simulink library "ece3413"  (R2018b)
settings: Solver=VariableStepAuto  StartTime=0.0  StopTime=10.0  RelTol=1e-3
settings Model: Creator=lbai  LastModifiedBy=bai

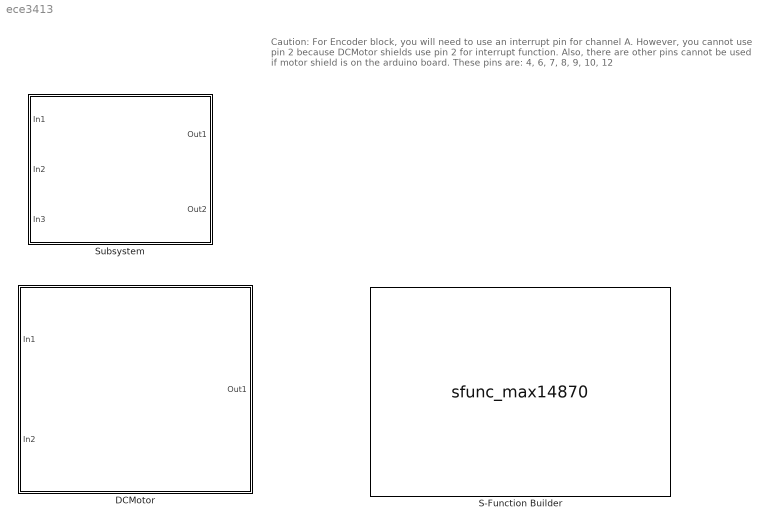
== system ece3413 ==
  note: Caution: For Encoder block, you will need to use an interrupt pin for channel A. However, you cannot use pin 2 because DCMotor shields use pin 2 for interrupt function. Also, there are other pins cannot be used if motor shield is on the arduino board. These pins are: 4, 6, 7, 8, 9, 10, 12
  DCMotor : Subsystem
      mask Display:
      | image('motor.jpg');
      | port_label('input', 1, 'motor#')
      | port_label('input', 2, 'speed')
      | port_label('output', 1, 'current')
  S-Function Builder : S-Function  InitFcn=try, set_param(gcb,'FunctionName','sfunc_max14870'), end  FunctionName=sfunc_max14870  SFunctionModules=sfunc_max14870_wrapper  SFunctionDeploymentMode=off  EnableBusSupport=off  mask(S-Function Builder){}
      mask help: Simulink:masks:SFunctionBuilder_MD
      mask init:
      | val = [[.9  0.75 0.75 1 1 .9 .9 1]',[1 1 0.75 0.75 .9 .9 1 .9]'];try , sys = get_param(gcb,'SfunBuilderFcnName');if isempty(sys), sys = get_param(gcb,'FunctionName'); end,catch, sys = get_param(gcb,'FunctionName'); end
      settings: CopyFcn=set_param(gcbh,'LinkStatus','none')  PreSaveFcn=try, set_param(gcb,'FunctionName','sfunc_max14870'), end  OpenFcn=sfunctionwizard(gcbh)
      mask Display:
      | image('smotor.jpg');
      | port_label('input', 1, 'motor#');
      | port_label('input', 2, 'motor pwm');
  Subsystem : Subsystem
      mask Display:
      | image('halleffect.jpg');
      | port_label('input', 1, 'A');
      | port_label('input', 2, 'B');
      | port_label('input', 3, 'sampleTIME');
      | port_label('output', 1, 'counter');
      | port_label('output', 2, 'rpm');

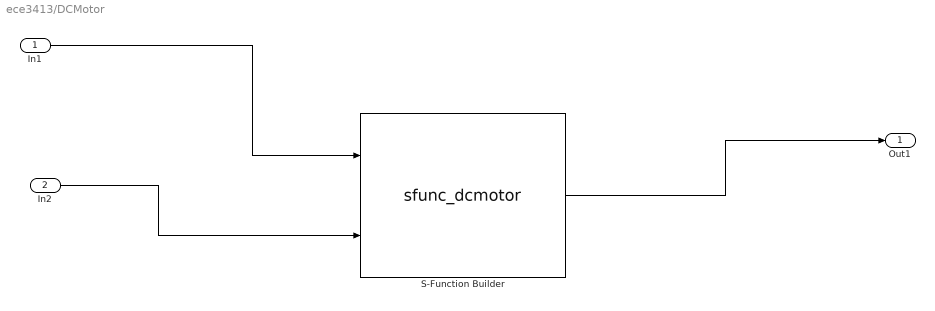
== system ece3413/DCMotor ==
  In1 : Inport
  In2 : Inport  Port=2
  S-Function Builder : S-Function  InitFcn=try, set_param(gcb,'FunctionName','sfunc_dcmotor'), end  FunctionName=sfunc_dcmotor  SFunctionModules=sfunc_dcmotor_wrapper  SFunctionDeploymentMode=off  EnableBusSupport=off  mask(S-Function Builder){}
      mask help: Simulink:masks:SFunctionBuilder_MD
      mask init: same as ece3413/S-Function Builder
      settings: CopyFcn=set_param(gcbh,'LinkStatus','none')  PreSaveFcn=try, set_param(gcb,'FunctionName','sfunc_dcmotor'), end  OpenFcn=sfunctionwizard(gcbh)
      mask Display: plot(val(:,1),val(:,2)),disp(sys), port_label('input',1,'mot'), port_label('input',2,'spd'), port_label('output',1,'current')
  Out1 : Outport
  wires:
  In2/1 -> S-Function Builder/2
  S-Function Builder/1 -> Out1/1
  In1/1 -> S-Function Builder/1

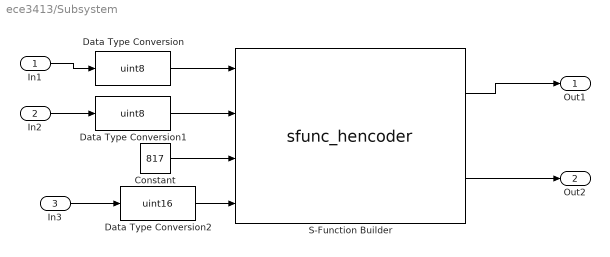
== system ece3413/Subsystem ==
  In1 : Inport
  In2 : Inport  Port=2
  In3 : Inport  Port=3
  Constant : Constant  Value=817  OutDataTypeStr=uint16
  Data Type Conversion : DataTypeConversion  OutDataTypeStr=uint8
  Data Type Conversion1 : DataTypeConversion  OutDataTypeStr=uint8
  Data Type Conversion2 : DataTypeConversion  OutDataTypeStr=uint16
  S-Function Builder : S-Function  InitFcn=try, set_param(gcb,'FunctionName','sfunc_hencoder'), end  FunctionName=sfunc_hencoder  SFunctionModules=sfunc_hencoder_wrapper  SFunctionDeploymentMode=off  EnableBusSupport=off  mask(S-Function Builder){}
      mask help: Simulink:masks:SFunctionBuilder_MD
      mask init: same as ece3413/S-Function Builder
      settings: CopyFcn=set_param(gcbh,'LinkStatus','none')  PreSaveFcn=try, set_param(gcb,'FunctionName','sfunc_hencoder'), end  OpenFcn=sfunctionwizard(gcbh)
      mask Display: plot(val(:,1),val(:,2)),disp(sys), port_label('input',1,'pinA'), port_label('input',2,'pinB'), port_label('input',3,'cntperrot'), port_label('input',4,'sampletime'), port_label('output',1,'pos'), port_label('output',2,'rpm')
  Out1 : Outport
  Out2 : Outport  Port=2
  wires:
  In3/1 -> Data Type Conversion2/1
  Data Type Conversion2/1 -> S-Function Builder/4
  In2/1 -> Data Type Conversion1/1
  Data Type Conversion1/1 -> S-Function Builder/2
  In1/1 -> Data Type Conversion/1
  Data Type Conversion/1 -> S-Function Builder/1
  Constant/1 -> S-Function Builder/3
  S-Function Builder/1 -> Out1/1
  S-Function Builder/2 -> Out2/1
